simulink model "inverse_dynamics2"  (R2024b)
settings: Solver=FixedStepAuto  StartTime=0.0  StopTime=tsim  FixedStep=dt  RelTol=1e-3
undefined symbols (not defined in the file or in its folder): f1, f2, h, Ix1, Iz1, Iz4, l1, l2, l3, l5, m1, m4, N1, N2, R, r, r1, r2, r3
settings Model: Creator=szymo  LastModifiedBy=mikol

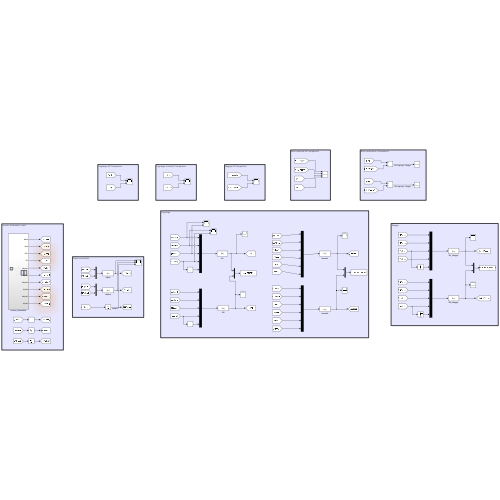
[thumbnail: Simulink's stored preview of the top-level diagram]
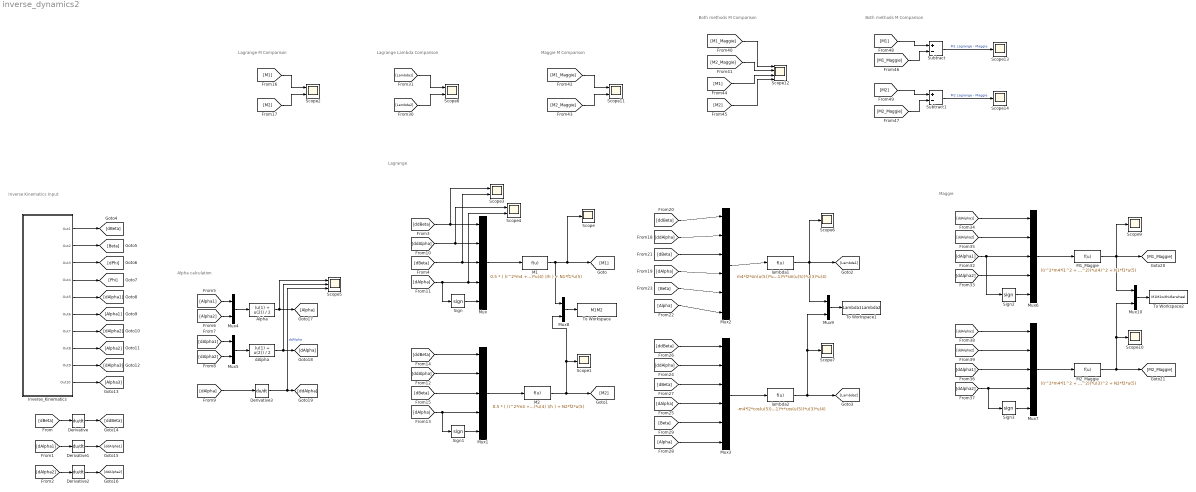
== system inverse_dynamics2 ==
  note: Maggie
  note: Lagrange
  note: Lagrange M Comparison
  note: Alpha calculation
  note: Inverse Kinematics Input
  note: Lagrange Lambda Comparison
  note: Maggie M Comparison
  note: Both methods M Comparison
  note: Both methods M Comparison
  Alpha : Fcn  Expr=(u(1) + u(2)) / 2
  Derivative{,1..3} (4 alike) : Derivative
  Inverse_Kinematics : Subsystem
  M1 : Fcn  Expr=0.5 * ( (r^2*m4 + 2*r^2*m1 +2*Iz1)*u(2) + m4*l2*u(3)^2 + ( (2*Iz1*h^2 + 2*m1*l1^2 + 2*Ix1 + Iz4 + m4*l2^2)*u(1) - m4*l2*r*u(3)*u(4) )/h ) + N1*f1*u(5)
  M1_Maggie : Fcn  Expr=((r^2*m4*l1^2 + 4*r^2*m1*l1^2 + 2*r^2*Ix1 + 4*Iz1*l1^2 + r^2*Iz4 + r^2*m4*l2^2) / (4*l1^2))*u(1) + ((r^2*m4*l1^2 - r^2*m4*l2^2 - 2*r^2*Ix1 - r^2*Iz4) / (4*l1^2))*u(2) - ((r^3*m4*l2) / (4*l1^2))*u(3)*u(4) + ((r^3*m4*l2) / (4*l1^2))*u(4)^2 + N1*f1*u(5)
  M2 : Fcn  Expr=0.5 * ( (r^2*m4 + 2*r^2*m1 +2*Iz1)*u(2) + m4*l2*u(3)^2 - ( (2*Iz1*h^2 + 2*m1*l1^2 + 2*Ix1 + Iz4 + m4*l2^2)*u(1) - m4*l2*r*u(3)*u(4) )/h ) + N2*f2*u(5)
  M2_Maggie : Fcn  Expr=((r^2*m4*l1^2 + 4*r^2*m1*l1^2 + 2*r^2*Ix1 + 4*Iz1*l1^2 + r^2*Iz4 + r^2*m4*l2^2) / (4*l1^2))*u(2) + ((r^2*m4*l1^2 - r^2*m4*l2^2 - 2*r^2*Ix1 - r^2*Iz4) / (4*l1^2))*u(1) - ((r^3*m4*l2) / (4*l1^2))*u(3)*u(4) + ((r^3*m4*l2) / (4*l1^2))*u(3)^2 + N2*f2*u(5)
  Mux{,1,6..7} (4 alike) : Mux  Inputs=5
  Mux{4..5,8..10} (5 alike) : Mux  Inputs=2
  Mux2 : Mux  Inputs=6
  Mux3 : Mux  Inputs=6
  Scope{,1,6..7,9..10,13..14} (8 alike) : Scope
  Scope{2..4,8,11} (5 alike) : Scope  NumInputPorts=2
  Scope12 : Scope  NumInputPorts=4
  Scope5 : Scope  NumInputPorts=3
  Sign{,1..3} (4 alike) : Signum
  Subtract : Sum  Inputs=+-
  Subtract1 : Sum  Inputs=+-
  To Workspace : ToWorkspace  VariableName=M1M2  SaveFormat=Timeseries  SampleTime=-1
  To Workspace1 : ToWorkspace  VariableName=Lambda1Lambda2  SaveFormat=Timeseries  SampleTime=-1
  To Workspace2 : ToWorkspace  VariableName=M1M2withidlerwheel  SaveFormat=Timeseries  SampleTime=-1
  dAlpha : Fcn  Expr=(u(1) + u(2)) / 2
  lambda1 : Fcn  Expr=m4*l2*sin(u(5))*u(1) + (m4 + 2*m1)*r*cos(u(5))*u(2) + m4*l2*cos(u(5))*u(3)^2 - (m4 +2*m1)*r*sin(u(5))*u(3)*u(4)
  lambda2 : Fcn  Expr=-m4*l2*cos(u(5))*u(1) + (m4 + 2*m1)*r*sin(u(5))*u(2) + m4*l2*sin(u(5))*u(3)^2 + (m4 +2*m1)*r*cos(u(5))*u(3)*u(4)
  wires:
  Mux/1 -> M1/1
  M1/1 -> Scope/1, [M1], Mux8/1
  M2/1 -> Scope1/1, Mux8/2, [M2]
  Inverse_Kinematics/1(Out1) -> [dBeta]
  Inverse_Kinematics/2(Out2) -> [Beta]
  Inverse_Kinematics/3(Out3) -> [dPhi]
  Inverse_Kinematics/4(Out4) -> [Phi]
  Inverse_Kinematics/5(Out5) -> [dAlpha1]
  Inverse_Kinematics/6(Out6) -> [Alpha1]
  Inverse_Kinematics/7(Out7) -> [dAlpha2]
  Inverse_Kinematics/8(Out8) -> [Alpha2]
  Inverse_Kinematics/9(Out9) -> [dAlpha3]
  Inverse_Kinematics/10(Out10) -> [Alpha3]
  [dBeta] -> Derivative/1
  [dAlpha1] -> Derivative1/1
  [dAlpha2] -> Derivative2/1
  Derivative/1 -> [ddBeta]
  Derivative1/1 -> [ddAlpha1]
  Derivative2/1 -> [ddAlpha2]
  Mux4/1 -> Alpha/1
  Mux5/1 -> dAlpha/1
  [Alpha1] -> Mux4/1
  [Alpha2] -> Mux4/2
  [dAlpha1] -> Mux5/1
  [dAlpha2] -> Mux5/2
  Alpha/1 -> [Alpha], Scope5/1
  dAlpha/1 -> [dAlpha], Scope5/2
  [dAlpha] -> Derivative3/1
  Derivative3/1 -> Scope5/3, [ddAlpha]  "ddAlpha"
  [ddBeta] -> Scope3/1, Mux/1
  [dBeta] -> Scope3/2, Mux/3
  [dAlpha] -> Sign/1, Scope4/2, Mux/4
  [ddAlpha] -> Scope4/1, Mux/2
  Sign/1 -> Mux/5
  [ddBeta] -> Mux1/1
  [ddAlpha] -> Mux1/2
  [dAlpha] -> Sign1/1, Mux1/4
  Sign1/1 -> Mux1/5
  [dBeta] -> Mux1/3
  Mux1/1 -> M2/1
  [M1] -> Scope2/1
  [M2] -> Scope2/2
  [dBeta] -> Mux2/3
  [ddAlpha] -> Mux2/2
  [ddBeta] -> Mux2/1
  Mux2/1 -> lambda1/1
  [dAlpha] -> Mux2/4
  lambda1/1 -> Scope6/1, [Lambda1], Mux9/1
  [Beta] -> Mux2/5
  [Alpha] -> Mux2/6
  [Beta] -> Mux3/5
  [dAlpha] -> Mux3/4
  [dBeta] -> Mux3/3
  [ddAlpha] -> Mux3/2
  [ddBeta] -> Mux3/1
  lambda2/1 -> [Lambda2], Mux9/2, Scope7/1
  [Alpha] -> Mux3/6
  Mux3/1 -> lambda2/1
  [Lambda2] -> Scope8/2
  [Lambda1] -> Scope8/1
  Mux6/1 -> M1_Maggie/1
  M1_Maggie/1 -> Mux10/1, Scope9/1, [M1_Maggie]
  Sign2/1 -> Mux6/5
  [ddAlpha1] -> Mux6/1
  [ddAlpha2] -> Mux6/2
  [dAlpha1] -> Sign2/1, Mux6/3
  [dAlpha2] -> Mux6/4
  Sign3/1 -> Mux7/5
  M2_Maggie/1 -> Mux10/2, Scope10/1, [M2_Maggie]
  Mux7/1 -> M2_Maggie/1
  [dAlpha2] -> Sign3/1, Mux7/4
  [ddAlpha2] -> Mux7/2
  [ddAlpha1] -> Mux7/1
  [dAlpha1] -> Mux7/3
  [M1_Maggie] -> Scope11/1
  [M2_Maggie] -> Scope11/2
  [M2_Maggie] -> Scope12/2
  [M1_Maggie] -> Scope12/1
  [M1] -> Scope12/3
  [M2] -> Scope12/4
  [M1] -> Subtract/1
  [M1_Maggie] -> Subtract/2
  [M2] -> Subtract1/1
  [M2_Maggie] -> Subtract1/2
  Subtract/1 -> Scope13/1  "M1 Lagrange - Maggie"
  Subtract1/1 -> Scope14/1  "M2 Lagrange - Maggie"
  Mux8/1 -> To Workspace/1
  Mux9/1 -> To Workspace1/1
  Mux10/1 -> To Workspace2/1

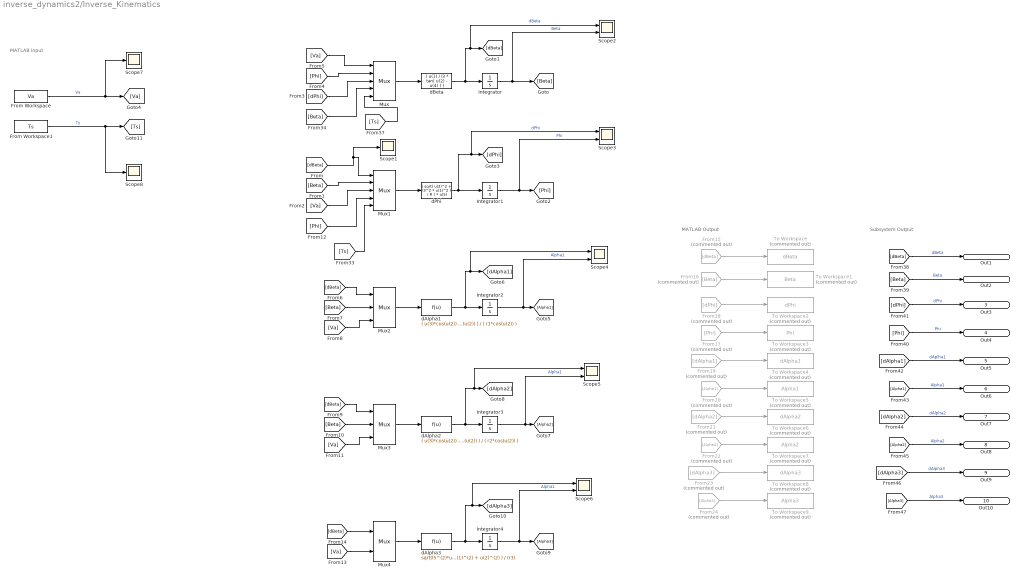
== system inverse_dynamics2/Inverse_Kinematics ==
  note: MATLAB Input
  note: MATLAB Output
  note: Subsystem Output
  From Workspace : FromWorkspace  VariableName=Va
  From Workspace1 : FromWorkspace  VariableName=Ts
  From15 : From  Commented=on  GotoTag=dBeta
  From16 : From  Commented=on  GotoTag=Beta
  From17 : From  Commented=on  GotoTag=Phi
  From18 : From  Commented=on  GotoTag=dPhi
  From19 : From  Commented=on  GotoTag=dAlpha1
  From20 : From  Commented=on  GotoTag=Alpha1
  From21 : From  Commented=on  GotoTag=dAlpha2
  From22 : From  Commented=on  GotoTag=Alpha2
  From23 : From  Commented=on  GotoTag=dAlpha3
  From24 : From  Commented=on  GotoTag=Alpha3
  Integrator{,1..4} (5 alike) : Integrator
  Mux : Mux  Inputs=5
      settings: DisplayOption=signals
  Mux1 : Mux  Inputs=5
      settings: DisplayOption=signals
  Mux2 : Mux  Inputs=3
      settings: DisplayOption=signals
  Mux3 : Mux  Inputs=3
      settings: DisplayOption=signals
  Mux4 : Mux  Inputs=2
      settings: DisplayOption=signals
  Scope1 : Scope
  Scope{2..6} (5 alike) : Scope  NumInputPorts=2
  Scope7 : Scope
  Scope8 : Scope
  To Workspace : ToWorkspace  Commented=on  VariableName=dBeta  SaveFormat=Timeseries  SampleTime=-1
  To Workspace1 : ToWorkspace  Commented=on  VariableName=Beta  SaveFormat=Timeseries  SampleTime=-1
  To Workspace2 : ToWorkspace  Commented=on  VariableName=dPhi  SaveFormat=Timeseries  SampleTime=-1
  To Workspace3 : ToWorkspace  Commented=on  VariableName=Phi  SaveFormat=Timeseries  SampleTime=-1
  To Workspace4 : ToWorkspace  Commented=on  VariableName=dAlpha1  SaveFormat=Timeseries  SampleTime=-1
  To Workspace5 : ToWorkspace  Commented=on  VariableName=Alpha1  SaveFormat=Timeseries  SampleTime=-1
  To Workspace6 : ToWorkspace  Commented=on  VariableName=dAlpha2  SaveFormat=Timeseries  SampleTime=-1
  To Workspace7 : ToWorkspace  Commented=on  VariableName=Alpha2  SaveFormat=Timeseries  SampleTime=-1
  To Workspace8 : ToWorkspace  Commented=on  VariableName=dAlpha3  SaveFormat=Timeseries  SampleTime=-1
  To Workspace9 : ToWorkspace  Commented=on  VariableName=Alpha3  SaveFormat=Timeseries  SampleTime=-1
  dAlpha1 : Fcn  Expr=( u(3)*cos(u(2)) + l1*u(1)*cos(u(2)) ) / ( r1*cos(u(2)) )
  dAlpha2 : Fcn  Expr=( u(3)*cos(u(2)) - l1*u(1)*cos(u(2)) ) / ( r2*cos(u(2)) )
  dAlpha3 : Fcn  Expr=sqrt(l5^(2)*u(1)^(2) + u(2)^(2) ) / (r3)
  dBeta : Fcn  Expr=( u(1) / l3 * tan( u(2) - u(4) ) )
  dPhi : Fcn  Expr="( sqrt( u(3)^2 + l3^2 * u(1)^2 ) / R )  * u(5)"
  Out1 : Outport
  Out2 : Outport  Port=2
  Out3 : Outport  Port=3
  Out4 : Outport  Port=4
  Out5 : Outport  Port=5
  Out6 : Outport  Port=6
  Out7 : Outport  Port=7
  Out8 : Outport  Port=8
  Out9 : Outport  Port=9
  Out10 : Outport  Port=10
  wires:
  From18/1 -> To Workspace2/1
  [Alpha1] -> Out6/1  "Alpha1"
  [Phi] -> Mux1/4
  [dBeta] -> Mux3/1
  [dAlpha2] -> Out7/1  "dAlpha2"
  From15/1 -> To Workspace/1
  [Va] -> Mux1/3
  Mux4/1 -> dAlpha3/1
  [Alpha3] -> Out10/1  "Alpha3"
  dPhi/1 -> Scope3/1, [dPhi], Integrator1/1  "dPhi"
  [dBeta] -> Out1/1  "dBeta"
  [dAlpha3] -> Out9/1  "dAlpha3"
  [Va] -> Mux2/3
  dBeta/1 -> Scope2/1, [dBeta], Integrator/1  "dBeta"
  [dPhi] -> Out3/1  "dPhi"
  From22/1 -> To Workspace7/1
  dAlpha3/1 -> Scope6/1, [dAlpha3], Integrator4/1
  [Va] -> Mux3/3
  [Phi] -> Out4/1  "Phi"
  From21/1 -> To Workspace6/1
  Integrator4/1 -> Scope6/2, [Alpha3]  "Alpha1"
  From17/1 -> To Workspace3/1
  From19/1 -> To Workspace4/1
  [dPhi] -> Mux/3
  [Beta] -> Mux/4
  [Beta] -> Out2/1  "Beta"
  Integrator2/1 -> Scope4/2, [Alpha1]  "Alpha1"
  Integrator1/1 -> Scope3/2, [Phi]  "Phi"
  [dAlpha1] -> Out5/1  "dAplha1"
  [Beta] -> Mux3/2
  From20/1 -> To Workspace5/1
  From24/1 -> To Workspace9/1
  From23/1 -> To Workspace8/1
  Mux3/1 -> dAlpha2/1
  From16/1 -> To Workspace1/1
  [dBeta] -> Mux2/1
  [Va] -> Mux4/2
  Mux1/1 -> dPhi/1
  Integrator/1 -> Scope2/2, [Beta]  "Beta"
  [Ts] -> Mux/5
  Mux/1 -> dBeta/1
  dAlpha1/1 -> Scope4/1, [dAlpha1], Integrator2/1
  From Workspace/1 -> Scope7/1, [Va]  "Va"
  Integrator3/1 -> Scope5/2, [Alpha2]  "Alpha1"
  dAlpha2/1 -> Scope5/1, [dAlpha2], Integrator3/1
  From Workspace1/1 -> Scope8/1, [Ts]  "Ts"
  [Ts] -> Mux1/5
  [dBeta] -> Scope1/1, Mux1/1
  [Alpha2] -> Out8/1  "Alpha2"
  [Beta] -> Mux1/2
  Mux2/1 -> dAlpha1/1
  [Beta] -> Mux2/2
  [Va] -> Mux/1
  [Phi] -> Mux/2
  [dBeta] -> Mux4/1
